simulink model "generate_command"  (Simulink 7.1)
settings: Solver=ode1  StartTime=0  StopTime=500  FixedStep=Ts  RelTol=1e-8
undefined symbols (not defined in the file or in its folder): command_on, psi_p_lim, x_p_lim, y_p_lim, z_p_lim
settings Model: Creator=Richard  LastModifiedBy=Richard  ExtModeTrigDuration=100
settings HardwareCC: ProdIntDivRoundTo=Zero  ProdEndianess=LittleEndian  ProdHWDeviceType=Intel->x86/Pentium  TargetBitPerLong=64  TargetEndianess=LittleEndian  TargetWordSize=64  TargetHWDeviceType=MATLAB Host  ProdEqTarget=off
settings RTWCC: SystemTargetFile=raccel.tlc  TemplateMakefile=raccel_default_tmf  RTWVerbose=off  ProcessScript=raccel_make_rtw_hook
settings CodeAppCC: GenerateComments=off  MaxIdLength=128  SimulinkBlockComments=off
settings RaccelTargetCC: TargetFunctionLibrary=ANSI_C  IsPILTarget=off  ERTFirstTimeCompliant=off  MultiInstanceERTCode=off  EnableShiftOperators=on  PortableWordSizes=off  ExtModeMexArgs='', 0, 61059  RTWCAPISignals=off  RTWCAPIParams=off

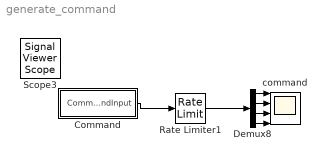
== system generate_command ==
  Command : Subsystem
  Demux8 : Demux
  Rate Limiter1 : RateLimiter  RisingSlewLimit=[x_p_lim y_p_lim z_p_lim psi_p_lim]  FallingSlewLimit=-[x_p_lim y_p_lim z_p_lim psi_p_lim]  SampleTimeMode=inherited
  command : Scope  NumInputPorts=4
      settings: TimeRange=25  YMin=9.5~-0.5~-0.1~-0.05  YMax=12~0.2000000000000001~0.6000000000000001~0.3  SaveName=command
  Scope3 : SignalViewerScope  IOType=viewer  NumInputPorts=4  RefreshTime=0.035000
  wires:
  Command/1(CommandInput) -> Rate Limiter1/1
  ? -> ?
  Demux8/1 -> command/1
  Demux8/2 -> command/2
  Demux8/3 -> command/3
  Demux8/4 -> command/4
  Rate Limiter1/1 -> Demux8/1

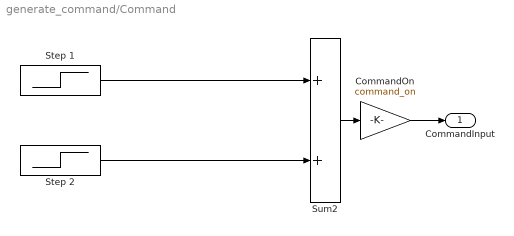
== system generate_command/Command ==
  CommandOn : Gain  Gain=command_on
  Step 1 : Step  Time=25  Before=zeros(1,4)  After="[24 24  -4 2]*1"  SampleTime=0
  Step 2 : Step  Time=70  Before=zeros(1,4)  After=[-24 -24 0 -2]*1  SampleTime=0
  Sum2 : Sum  Inputs=2
  CommandInput : Outport
  wires:
  Step 1/1 -> Sum2/1
  Sum2/1 -> CommandOn/1
  Step 2/1 -> Sum2/2
  CommandOn/1 -> CommandInput/1
